simulink model "malha_aberta"  (R2013a)
settings: Solver=ode45  SolverMode=SingleTasking  StartTime=0.0  StopTime=10.0  RelTol=1e-3
values from neighbouring files (symbols this model uses):
  C = 200    [Exercicio3.m]    (also in setup.m = 0.0008)
  D = 0.3    [setup.m]
  L = 1/1000    (= 0.001)    [setup.m]
  R = 1    [setup.m]
  Vi = 1    [setup.m]
settings Model: Creator=05630646761  LastModifiedBy=05630646761
settings DataIOCC: SignalLoggingSaveFormat=ModelDataLogs
settings OptimizationCC: BlockReduction=off  BooleanDataType=off
settings DebuggingCC: SaveWithParameterizedLinksMsg=none  SignalResolutionControl=TryResolveAllWithWarning  SolverPrmCheckMsg=none  MultiTaskDSMMsg=warning  MultiTaskCondExecSysMsg=none  StrictBusMsg=None
settings HardwareCC: TargetUnknown=on
settings RTWCC: IncludeERTFirstTime=on

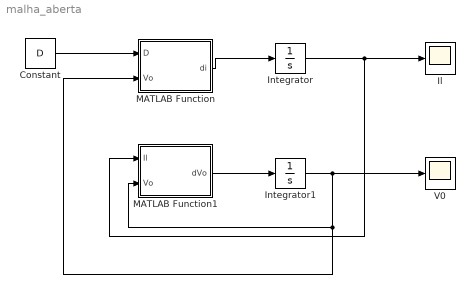
== system malha_aberta ==
  Constant : Constant  Value=D
  Il : Scope
  Integrator : Integrator
  Integrator1 : Integrator
  MATLAB Function : MATLAB Function  TreatAsAtomicUnit=on
  MATLAB Function1 : MATLAB Function  TreatAsAtomicUnit=on
  V0 : Scope
  wires:
  MATLAB Function/1(di) -> Integrator/1
  MATLAB Function1/1(dVo) -> Integrator1/1
  Integrator1/1 -> MATLAB Function1/2(Vo), MATLAB Function/2(Vo), V0/1
  Integrator/1 -> MATLAB Function1/1(Il), Il/1
  Constant/1 -> MATLAB Function/1(D)

== matlab function malha_aberta/MATLAB Function1 ==
  data: Il input; dVo output; Vo input; R parameter; C parameter
function dVo = fcn(Il, Vo, R, C)

dVo = Il/C - Vo/(R*C) ;

== matlab function malha_aberta/MATLAB Function ==
  data: D input; di output; Vi parameter; Vo input; L parameter
function di = fcn(D, Vi, Vo, L)

di = D*Vi/Vo - Vo/L;
